simulink model "Six_quad_formation_100714"  (R2012b)
settings: Solver=ode5  StartTime=0.0  StopTime=inf  FixedStep=sample_time  RelTol=1e-3
InitFcn:
  | sample_time=0.005;%0.004;%0.0025;%0.02;
  | sample_time_Vicon = 0.005;
  | DeltaT = 0.02;
  | g = 9.81;
  | H0 = g%0.3165;
  | Kl = 1;
  | 
  | Q6_mass = 0.8;
  | 
  | Q6_Omega_r = 1.2; %for horizon ref
  | Q6_Zeta_r = 0.707; %for horizon ref
  | Q6_Omega_r_h = 2;%for vertical ref
  | Q6_Zeta_r_h = 0.7; %for vertical ref
  | 
  | 
  | Q6_Omega = 1.5; %for horizon control
  | Q6_Zeta = 0.507; %for horizon control
  | Q6_Omega_h= 2 %for vertical control
  | Q6_Zeta_h = 0.5; %for vertical control
  | 
  | 
  | Q6_acc_max = 5;%horizontal max acc
  | Q6_acc_max_h = 5;%horizontal max acc
  | 
  | omega_circle = 10*pi/180;
  | 
  | omega_h = 0.1;%Ascending speed
  | PI = pi;
  | Circle_R = 2;
  | 
  | 
  | MAX_Height = -2;
  | 
  | 
  | % for NN
  | n = 5;
  | r = 3;
  | n2 = 5;
  | NN_ST = 0.02;
  | 
  | GAMA_V = 6;
  | gama_V_e = 0.01;
  | 
  | GAMA_W = GAMA_V;
  | gama_W_e =0.01;
  | 
  | % deadzone
  | NN_Deadzone_Z = 0;
  | 
  | % inputs nomalizaton parameters
  | NN_Z_y_min = -3;
  | NN_Z_y_max = 0.5;
  | 
  | NN_Z_v_max = 8;
  | NN_Z_v_min = -NN_Z_v_max;
  | 
  | % alpha = 0.034;
  | alpha = 1;
  | % c_f = 0.0015;
  | c_f = 0.001;
  | ... (+1 lines)
libraries: X330_Control x30, simulink x12
(part 2 of 2)

== system Six_quad_formation_100714/Vicon_Data/Raw Quad Pose from Vicon/Process Vicon Raw Data1/Flip_pi1/Flip_0_to_2pi/Flip_2pi ==
  Angle : Inport
  Bias : Bias  Bias=-2*pi
  Constant : Constant  Value=2*pi
  Data Type Duplicate : DataTypeDuplicate
  Modulo : Math  Operator=mod  SaturateOnIntegerOverflow=on
  Sign1 : Signum
  Switch : Switch
  Angle_Flip : Outport
  wires:
  Switch/1 -> Data Type Duplicate/2, Angle_Flip/1
  Bias/1 -> Switch/3
  Sign1/1 -> Switch/2
  Modulo/1 -> Switch/1, Bias/1
  Constant/1 -> Modulo/2
  Angle/1 -> Data Type Duplicate/1, Sign1/1, Modulo/1

== system Six_quad_formation_100714/Vicon_Data/Raw Quad Pose from Vicon/Process Vicon Raw Data2/Flip_pi1/Flip_0_to_2pi/Flip_2pi ==
  Angle : Inport
  Bias : Bias  Bias=-2*pi
  Constant : Constant  Value=2*pi
  Data Type Duplicate : DataTypeDuplicate
  Modulo : Math  Operator=mod  SaturateOnIntegerOverflow=on
  Sign1 : Signum
  Switch : Switch
  Angle_Flip : Outport
  wires:
  Angle/1 -> Modulo/1, Sign1/1, Data Type Duplicate/1
  Constant/1 -> Modulo/2
  Modulo/1 -> Bias/1, Switch/1
  Sign1/1 -> Switch/2
  Bias/1 -> Switch/3
  Switch/1 -> Angle_Flip/1, Data Type Duplicate/2

== system Six_quad_formation_100714/Vicon_Data/Raw Quad Pose from Vicon/Process Vicon Raw Data3/Flip_pi1/Flip_0_to_2pi/Flip_2pi ==
  Angle : Inport
  Bias : Bias  Bias=-2*pi
  Constant : Constant  Value=2*pi
  Data Type Duplicate : DataTypeDuplicate
  Modulo : Math  Operator=mod  SaturateOnIntegerOverflow=on
  Sign1 : Signum
  Switch : Switch
  Angle_Flip : Outport
  wires:
  Angle/1 -> Modulo/1, Sign1/1, Data Type Duplicate/1
  Constant/1 -> Modulo/2
  Modulo/1 -> Bias/1, Switch/1
  Sign1/1 -> Switch/2
  Bias/1 -> Switch/3
  Switch/1 -> Angle_Flip/1, Data Type Duplicate/2

== system Six_quad_formation_100714/Vicon_Data/Raw Quad Pose from Vicon/Process Vicon Raw Data4/Flip_pi1/Flip_0_to_2pi/Flip_2pi ==
  Angle : Inport
  Bias : Bias  Bias=-2*pi
  Constant : Constant  Value=2*pi
  Data Type Duplicate : DataTypeDuplicate
  Modulo : Math  Operator=mod  SaturateOnIntegerOverflow=on
  Sign1 : Signum
  Switch : Switch
  Angle_Flip : Outport
  wires:
  Switch/1 -> Data Type Duplicate/2, Angle_Flip/1
  Bias/1 -> Switch/3
  Sign1/1 -> Switch/2
  Modulo/1 -> Switch/1, Bias/1
  Constant/1 -> Modulo/2
  Angle/1 -> Data Type Duplicate/1, Sign1/1, Modulo/1

== system Six_quad_formation_100714/Vicon_Data/Raw Quad Pose from Vicon/Process Vicon Raw Data5/Flip_pi1/Flip_0_to_2pi/Flip_2pi ==
  Angle : Inport
  Bias : Bias  Bias=-2*pi
  Constant : Constant  Value=2*pi
  Data Type Duplicate : DataTypeDuplicate
  Modulo : Math  Operator=mod  SaturateOnIntegerOverflow=on
  Sign1 : Signum
  Switch : Switch
  Angle_Flip : Outport
  wires:
  Switch/1 -> Data Type Duplicate/2, Angle_Flip/1
  Bias/1 -> Switch/3
  Sign1/1 -> Switch/2
  Modulo/1 -> Switch/1, Bias/1
  Constant/1 -> Modulo/2
  Angle/1 -> Data Type Duplicate/1, Sign1/1, Modulo/1

== system Six_quad_formation_100714/Vicon_Data/Raw Quad Pose from Vicon/Process Vicon Raw Data6/Flip_pi1/Flip_0_to_2pi/Flip_2pi ==
  Angle : Inport
  Bias : Bias  Bias=-2*pi
  Constant : Constant  Value=2*pi
  Data Type Duplicate : DataTypeDuplicate
  Modulo : Math  Operator=mod  SaturateOnIntegerOverflow=on
  Sign1 : Signum
  Switch : Switch
  Angle_Flip : Outport
  wires:
  Angle/1 -> Modulo/1, Sign1/1, Data Type Duplicate/1
  Constant/1 -> Modulo/2
  Modulo/1 -> Bias/1, Switch/1
  Sign1/1 -> Switch/2
  Bias/1 -> Switch/3
  Switch/1 -> Angle_Flip/1, Data Type Duplicate/2

== stateflow chart Six_quad_formation_100714/Subsystem/Trajectory Logic/ SF ==
  state Airborne
    state TakeOff
      du:		HoverThrottle = (H0 - HoverThrottle)*2*DeltaT + HoverThrottle ;
      PosDes_UAV1[2] = (-1.2 - PosDes_UAV1[2])*1*DeltaT + PosDes_UAV1[2] ;
      PosDes_UAV2[2] = (-1.2 - PosDes_UAV2[2])*1*DeltaT + PosDes_UAV2[2] ;
      PosDes_UAV3[2] = (-1.2 - PosDes_UAV3[2])*1*DeltaT + PosDes_UAV3[2] ;
      PosDes_UAV4[2] = (-1.2 - PosDes_UAV4[2])*1*DeltaT + PosDes_UAV4[2] ;
      PosDes_UAV5[2] = (-1.2 - PosDes_UAV5[2])*1*DeltaT + PosDes_UAV5[2] ;
      PosDes_UAV6[2] = (-1.2 - PosDes_UAV6[2])*1*DeltaT + PosDes_UAV6[2] ;
    state Stage1
      state Red_UAV1 [parallel]
        du:PosDes_UAV1[0] = (-2- PosDes_UAV1[0])*0.5*DeltaT + PosDes_UAV1[0] ;
        PosDes_UAV1[1] = (2- PosDes_UAV1[1])*0.5*DeltaT + PosDes_UAV1[1] ;
        PosDes_UAV1[2] = (-1.2- PosDes_UAV1[2])*0.5*DeltaT + PosDes_UAV1[2] ;
        settings: executionOrder=1
      state Green_UAV2 [parallel]
        du:PosDes_UAV2[0] = (-2-PosDes_UAV2[0])*0.5*DeltaT+PosDes_UAV2[0];
        PosDes_UAV2[1] = (1-PosDes_UAV2[1])*0.5*DeltaT+PosDes_UAV2[1];
        PosDes_UAV2[2] = (-1.2-PosDes_UAV2[2])*0.5*DeltaT+PosDes_UAV2[2];
        settings: executionOrder=2
      state PWM [parallel]
        du:    pwm=  1800;
        settings: executionOrder=3
      state Blue_UAV3 [parallel]
        du:PosDes_UAV3[0] = (-2-PosDes_UAV3[0])*0.5*DeltaT + PosDes_UAV3[0];
        PosDes_UAV3[1] = (0-PosDes_UAV3[1])*0.5*DeltaT+PosDes_UAV3[1];
        PosDes_UAV3[2] = (-1.2-PosDes_UAV3[2])*0.5*DeltaT+PosDes_UAV3[2];
        settings: executionOrder=4
      state Purple_UAV4 [parallel]
        du:PosDes_UAV4[0] = (-2-PosDes_UAV4[0])*0.5*DeltaT + PosDes_UAV4[0];
        PosDes_UAV4[1] = (-1-PosDes_UAV4[1])*0.5*DeltaT+PosDes_UAV4[1];
        PosDes_UAV4[2] = (-1.2-PosDes_UAV4[2])*0.5*DeltaT+PosDes_UAV4[2];
        settings: executionOrder=5
      state Purple_UAV5 [parallel]
        du:PosDes_UAV5[0] = (-2-PosDes_UAV5[0])*0.5*DeltaT + PosDes_UAV5[0];
        PosDes_UAV5[1] = (-2-PosDes_UAV5[1])*0.5*DeltaT+PosDes_UAV5[1];
        PosDes_UAV5[2] = (-1.2-PosDes_UAV5[2])*0.5*DeltaT+PosDes_UAV5[2];
        settings: executionOrder=6
      state Purple_UAV6 [parallel]
        du:PosDes_UAV6[0] = (-2-PosDes_UAV6[0])*0.5*DeltaT + PosDes_UAV6[0];
        PosDes_UAV6[1] = (-3-PosDes_UAV6[1])*0.5*DeltaT+PosDes_UAV6[1];
        PosDes_UAV6[2] = (-1.2-PosDes_UAV6[2])*0.5*DeltaT+PosDes_UAV6[2];
        settings: executionOrder=7
    state Stage2
      state Red_UAV1 [parallel]
        du:PosDes_UAV1[0] = (0- PosDes_UAV1[0])*0.5*DeltaT + PosDes_UAV1[0] ;
        PosDes_UAV1[1] = (2- PosDes_UAV1[1])*0.5*DeltaT + PosDes_UAV1[1] ;
        PosDes_UAV1[2] = (-1.2- PosDes_UAV1[2])*0.5*DeltaT + PosDes_UAV1[2] ;
        settings: executionOrder=1
      state Green_UAV2 [parallel]
        du:PosDes_UAV2[0] = (0-PosDes_UAV2[0])*0.5*DeltaT+PosDes_UAV2[0];
        PosDes_UAV2[1] = (1-PosDes_UAV2[1])*0.5*DeltaT+PosDes_UAV2[1];
        PosDes_UAV2[2] = (-1.2-PosDes_UAV2[2])*0.5*DeltaT+PosDes_UAV2[2];
        settings: executionOrder=2
      state PWM [parallel]
        du:    pwm=  1800;
        settings: executionOrder=3
      state Blue_UAV3 [parallel]
        du:PosDes_UAV3[0] = (0-PosDes_UAV3[0])*0.5*DeltaT + PosDes_UAV3[0];
        PosDes_UAV3[1] = (0-PosDes_UAV3[1])*0.5*DeltaT+PosDes_UAV3[1];
        PosDes_UAV3[2] = (-1.2-PosDes_UAV3[2])*0.5*DeltaT+PosDes_UAV3[2];
        settings: executionOrder=4
      state Purple_UAV4 [parallel]
        du:PosDes_UAV4[0] = (0-PosDes_UAV4[0])*0.5*DeltaT + PosDes_UAV4[0];
        PosDes_UAV4[1] = (-1-PosDes_UAV4[1])*0.5*DeltaT+PosDes_UAV4[1];
        PosDes_UAV4[2] = (-1.2-PosDes_UAV4[2])*0.5*DeltaT+PosDes_UAV4[2];
        settings: executionOrder=5
      state Purple_UAV5 [parallel]
        du:PosDes_UAV5[0] = (0-PosDes_UAV5[0])*0.5*DeltaT + PosDes_UAV5[0];
        PosDes_UAV5[1] = (-2-PosDes_UAV5[1])*0.5*DeltaT+PosDes_UAV5[1];
        PosDes_UAV5[2] = (-1.2-PosDes_UAV5[2])*0.5*DeltaT+PosDes_UAV5[2];
        settings: executionOrder=6
      state Purple_UAV6 [parallel]
        du:PosDes_UAV6[0] = (0-PosDes_UAV6[0])*0.5*DeltaT + PosDes_UAV6[0];
        PosDes_UAV6[1] = (-3-PosDes_UAV6[1])*0.5*DeltaT+PosDes_UAV6[1];
        PosDes_UAV6[2] = (-1.2-PosDes_UAV6[2])*0.5*DeltaT+PosDes_UAV6[2];
        settings: executionOrder=7
    (default) -> TakeOff : {	PosDes_UAV1 = Pos_UAV1;
        | 	PosDes_UAV2 = Pos_UAV2;
        | 	PosDes_UAV3 = Pos_UAV3;
        | 	PosDes_UAV4 = Pos_UAV4;
        | 	PosDes_UAV5 = Pos_UAV5;
        | 	PosDes_UAV6 = Pos_UAV6;
        | 	 }
    TakeOff -> Stage1 : after (3, sec)
    Stage1 -> (junction 637) : after (15,sec)
    (junction 639) -> Stage1 : [abs(Pos_UAV1[0]-0)<0.1]
    (junction 637) -> Stage2 : [abs(Pos_UAV1[0]-(-2))<0.1]
    Stage2 -> (junction 639) : after (15,sec)
  state Landing
    state Decsending
      en:		PosDes_UAV1 = Pos_UAV1;	PosDes_UAV2 = Pos_UAV2;  PosDes_UAV3 = Pos_UAV3;
      PosDes_UAV4 = Pos_UAV4;  PosDes_UAV5 = Pos_UAV5;  PosDes_UAV6 = Pos_UAV6;
      du:		PosDes_UAV1[2] = (0 - PosDes_UAV1[2])*0.2*DeltaT + PosDes_UAV1[2] ;
      PosDes_UAV2[2] = (0 - PosDes_UAV2[2])*0.2*DeltaT + PosDes_UAV2[2] ;
      PosDes_UAV3[2] = (0 - PosDes_UAV3[2])*0.2*DeltaT + PosDes_UAV3[2] ;
      PosDes_UAV4[2] = (0 - PosDes_UAV4[2])*0.2*DeltaT + PosDes_UAV4[2] ;
      PosDes_UAV5[2] = (0 - PosDes_UAV5[2])*0.2*DeltaT + PosDes_UAV5[2] ;
      PosDes_UAV6[2] = (0 - PosDes_UAV6[2])*0.2*DeltaT + PosDes_UAV6[2] ;
    state CutThrottle
      du:		HoverThrottle = (0.0 - HoverThrottle)*3*DeltaT + HoverThrottle ;
    (default) -> Decsending
    Decsending -> (junction 288) : after(2,sec)
    (junction 288) -> CutThrottle : [Pos_UAV1[2] > -0.2]
  Landing -> Airborne : [RC[6] > 0.5]
  Airborne -> Landing : [RC[6] < -0.5]
  (default) -> Landing : {HoverThrottle=0.0}
  data: HoverThrottle output double size=1; PosDes_UAV1 output double size=4; PosDes_UAV2 output double size=4; PosDes_UAV3 output double size=4; RC input size=8; Pos_UAV1 input size=4; DeltaT parameter size=1; H0 parameter size=1; Kl parameter size=1; Increm local double size=1; omega_circle parameter size=1; PI parameter size=1; omega_h parameter; Circle_R parameter size=1; MAX_Height parameter size=1; Pos_UAV2 input size=4; Pos_UAV3 input size=4; Pos_UAV4 input size=4; PosDes_UAV4 output double size=4; Pos_UAV5 input size=4; Pos_UAV6 input size=4; PosDes_UAV5 output double size=4; PosDes_UAV6 output double size=4; pwm output double
